simulink model "Aero_UltraStick25e"  (R2016b)
settings: Solver=VariableStepAuto  StartTime=0.0  StopTime=10.0  RelTol=1e-3
undefined symbols (not defined in the file or in its folder): AC
libraries: simulink x1
(part 1 of 2)
settings Model: Creator=UAVLAB  LastModifiedBy=UAVLAB

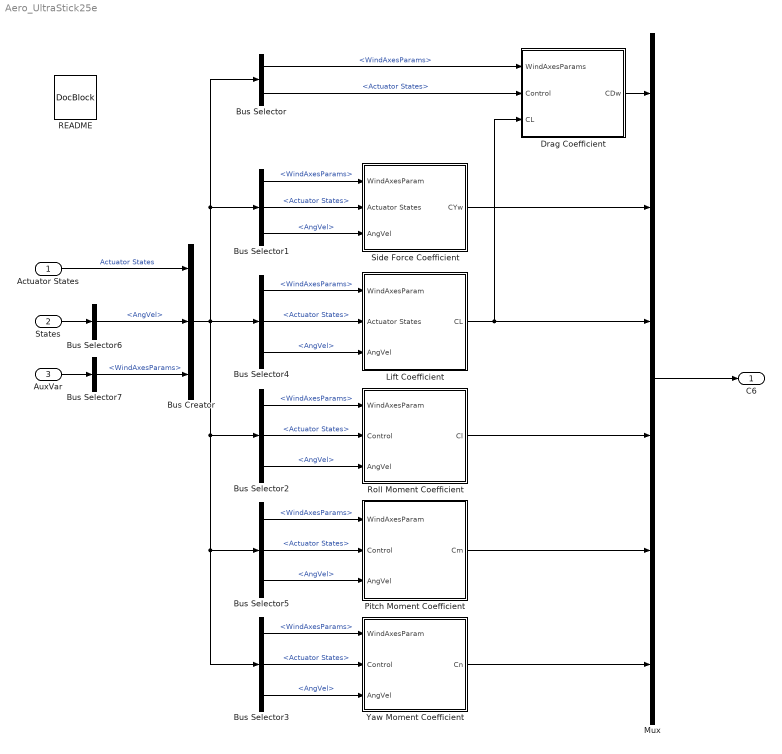
== system Aero_UltraStick25e ==
  Actuator States : Inport  OutDataTypeStr=Bus: Actuators
  States : Inport  Port=2  OutDataTypeStr=Bus: RigidStates
  AuxVar : Inport  Port=3  OutDataTypeStr=Bus: AuxVar
  Bus Creator : BusCreator  Inputs=3
  Bus Selector : BusSelector  OutputSignals=WindAxesParams,Actuator States
  Bus Selector{1..5} (5 alike) : BusSelector  OutputSignals=WindAxesParams,Actuator States,AngVel
  Bus Selector6 : BusSelector  OutputSignals=AngVel
  Bus Selector7 : BusSelector  OutputSignals=WindAxesParams
  Drag Coefficient : Subsystem
  Lift Coefficient : Subsystem
  Mux : Mux  Inputs=6
  Pitch Moment Coefficient : Subsystem
  README : simulink/Model-Wide Utilities/DocBlock  DocumentType=Text
      content=|
      | Ultrastick Aerodynamic Model
      |
      | This block models the Ultrastick aerodynamics using a linear derivatives.
      | The force coefficients are in the wind axes, but the moment coefficients
      | are in body axes, so the six coefficients are CL, CDw, CYw, Cl, Cm, Cn.
      | See Klein, Morelli, Aircraft System Identification, pg 41. Thus in the
      | Aero lib, the force and moment transformation block must be set as though
      | outgoing moment coefficients are in wind axes so no transformation is
      | applied.
      |
      | The derivatives are stored in the aircraft configuration data structure
      | (AC). They are loaded into AC.Aero when 'Ulstrastick' is selected with
      | UAV_config.m.  The derivatives themselves are stored in
      | Ultrastick_config.m. An example is the derivatives for CL:
      |
      | >>  AC.Aero.CL
      |
      | ans =
      |
      |         zero: 0.1086
      |        alpha: 4.5800
      |        dflap: 0.7400
      |        delev: 0.0983
      |     alphadot: 1.9724
      |            q: 6.1639
      |         minD: 0.2300
      |
      | The majority of the derivatives have been indentified from flight test
      | data. The drag model was derived from first principles.
  Roll Moment Coefficient : Subsystem
  Side Force Coefficient : Subsystem
  Yaw Moment Coefficient : Subsystem
  C6 : Outport
  wires:
  Bus Selector/2 -> Drag Coefficient/2(Control)  "<Actuator States>"
  Bus Selector5/3 -> Pitch Moment Coefficient/3(AngVel)  "<AngVel>"
  Bus Selector5/2 -> Pitch Moment Coefficient/2(Control)  "<Actuator States>"
  Bus Selector5/1 -> Pitch Moment Coefficient/1(WindAxesParam)  "<WindAxesParams>"
  Bus Selector4/3 -> Lift Coefficient/3(AngVel)  "<AngVel>"
  Bus Selector4/2 -> Lift Coefficient/2(Actuator States)  "<Actuator States>"
  Bus Selector4/1 -> Lift Coefficient/1(WindAxesParam)  "<WindAxesParams>"
  Bus Selector3/3 -> Yaw Moment Coefficient/3(AngVel)  "<AngVel>"
  Bus Selector3/2 -> Yaw Moment Coefficient/2(Control)  "<Actuator States>"
  Bus Selector3/1 -> Yaw Moment Coefficient/1(WindAxesParam)  "<WindAxesParams>"
  Bus Selector2/3 -> Roll Moment Coefficient/3(AngVel)  "<AngVel>"
  Bus Selector2/2 -> Roll Moment Coefficient/2(Control)  "<Actuator States>"
  Bus Selector2/1 -> Roll Moment Coefficient/1(WindAxesParam)  "<WindAxesParams>"
  Bus Selector1/3 -> Side Force Coefficient/3(AngVel)  "<AngVel>"
  Bus Selector1/2 -> Side Force Coefficient/2(Actuator States)  "<Actuator States>"
  Bus Selector1/1 -> Side Force Coefficient/1(WindAxesParam)  "<WindAxesParams>"
  Bus Creator/1 -> Bus Selector1/1, Bus Selector/1, Bus Selector4/1, Bus Selector5/1, Bus Selector3/1, Bus Selector2/1
  Mux/1 -> C6/1
  Yaw Moment Coefficient/1(Cn) -> Mux/6
  Pitch Moment Coefficient/1(Cm) -> Mux/5
  Roll Moment Coefficient/1(Cl) -> Mux/4
  Side Force Coefficient/1(CYw) -> Mux/2
  Drag Coefficient/1(CDw) -> Mux/1
  States/1 -> Bus Selector6/1
  Bus Selector6/1 -> Bus Creator/2  "<AngVel>"
  Lift Coefficient/1(CL) -> Mux/3, Drag Coefficient/3(CL)
  AuxVar/1 -> Bus Selector7/1
  Bus Selector7/1 -> Bus Creator/3  "<WindAxesParams>"
  Actuator States/1 -> Bus Creator/1  "Actuator States"
  Bus Selector/1 -> Drag Coefficient/1(WindAxesParams)  "<WindAxesParams>"

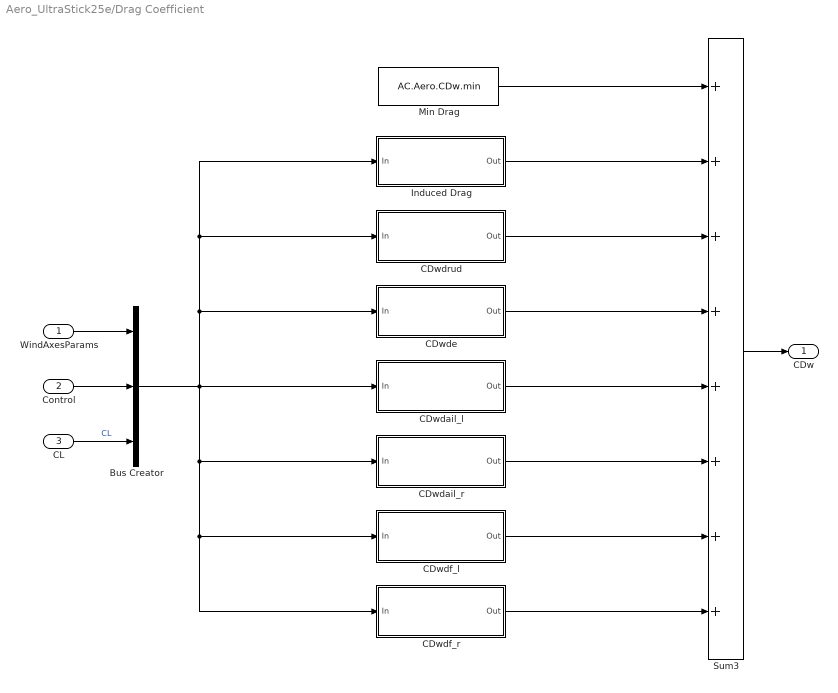
== system Aero_UltraStick25e/Drag Coefficient ==
  WindAxesParams : Inport
  Control : Inport  Port=2
  CL : Inport  Port=3
  Bus Creator : BusCreator  Inputs=3
  CDwdail_l : Subsystem
  CDwdail_r : Subsystem
  CDwde : Subsystem
  CDwdf_l : Subsystem
  CDwdf_r : Subsystem
  CDwdrud : Subsystem
  Induced Drag : Subsystem
  Min Drag : Constant  Value=AC.Aero.CDw.min
  Sum3 : Sum  Inputs=++++++++  SaturateOnIntegerOverflow=on  InputSameDT=on  OutDataTypeStr=Inherit: Same as first input
  CDw : Outport
  wires:
  Min Drag/1 -> Sum3/1
  CDwdrud/1(Out) -> Sum3/3
  CDwde/1(Out) -> Sum3/4
  CDwdail_l/1(Out) -> Sum3/5
  CDwdail_r/1(Out) -> Sum3/6
  CDwdf_l/1(Out) -> Sum3/7
  CDwdf_r/1(Out) -> Sum3/8
  Sum3/1 -> CDw/1
  Bus Creator/1 -> CDwdail_l/1(In), CDwdrud/1(In), Induced Drag/1(In), CDwde/1(In), CDwdail_r/1(In), CDwdf_l/1(In), CDwdf_r/1(In)
  Induced Drag/1(Out) -> Sum3/2
  WindAxesParams/1 -> Bus Creator/1
  Control/1 -> Bus Creator/2
  CL/1 -> Bus Creator/3  "CL"

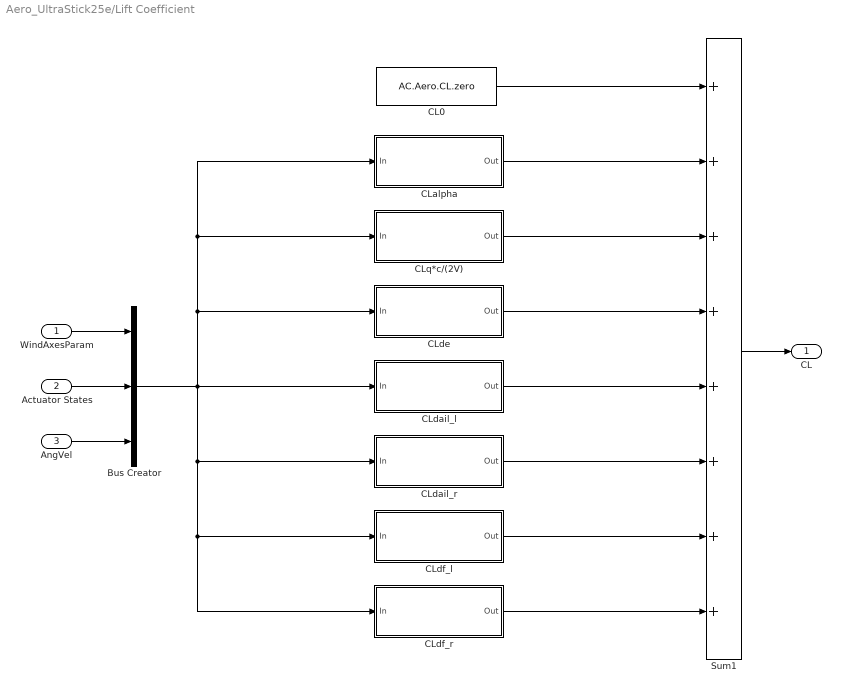
== system Aero_UltraStick25e/Lift Coefficient ==
  WindAxesParam : Inport
  Actuator States : Inport  Port=2  OutDataTypeStr=Bus: Actuators
  AngVel : Inport  Port=3
  Bus Creator : BusCreator  Inputs=3
  CL0 : Constant  Value=AC.Aero.CL.zero
  CLalpha : Subsystem
  CLdail_l : Subsystem
  CLdail_r : Subsystem
  CLde : Subsystem
  CLdf_l : Subsystem
  CLdf_r : Subsystem
  CLq*c/(2V) : Subsystem
  Sum1 : Sum  Inputs=++++++++  SaturateOnIntegerOverflow=on  InputSameDT=on  OutDataTypeStr=Inherit: Same as first input
  CL : Outport
  wires:
  WindAxesParam/1 -> Bus Creator/1
  Actuator States/1 -> Bus Creator/2
  AngVel/1 -> Bus Creator/3
  Bus Creator/1 -> CLdail_l/1(In), CLalpha/1(In), CLq*c/(2V)/1(In), CLde/1(In), CLdail_r/1(In), CLdf_l/1(In), CLdf_r/1(In)
  CLalpha/1(Out) -> Sum1/2
  CL0/1 -> Sum1/1
  CLq*c/(2V)/1(Out) -> Sum1/3
  CLde/1(Out) -> Sum1/4
  CLdail_l/1(Out) -> Sum1/5
  CLdail_r/1(Out) -> Sum1/6
  CLdf_l/1(Out) -> Sum1/7
  CLdf_r/1(Out) -> Sum1/8
  Sum1/1 -> CL/1

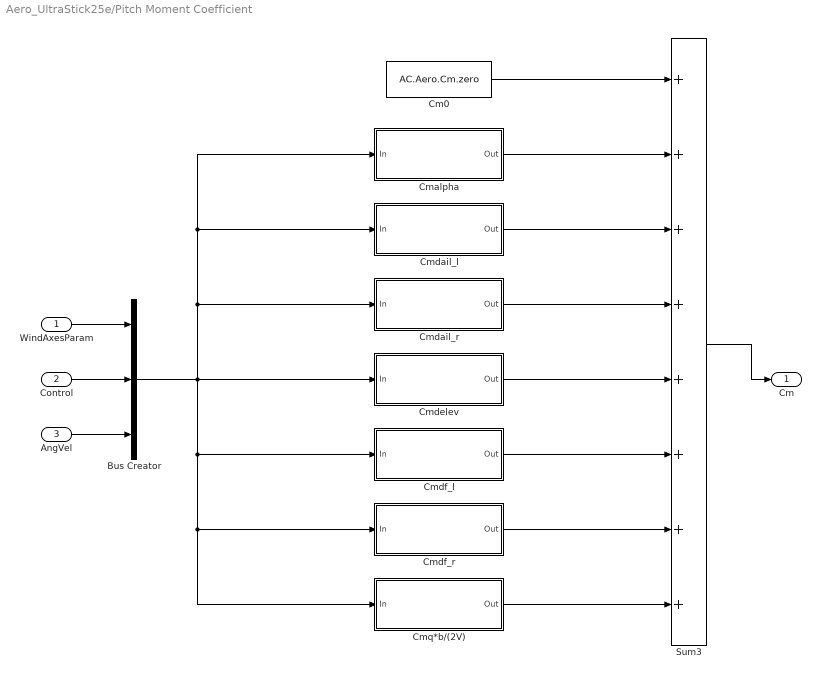
== system Aero_UltraStick25e/Pitch Moment Coefficient ==
  WindAxesParam : Inport
  Control : Inport  Port=2
  AngVel : Inport  Port=3
  Bus Creator : BusCreator  Inputs=3
  Cm0 : Constant  Value=AC.Aero.Cm.zero
  Cmalpha : Subsystem
  Cmdail_l : Subsystem
  Cmdail_r : Subsystem
  Cmdelev : Subsystem
  Cmdf_l : Subsystem
  Cmdf_r : Subsystem
  Cmq*b/(2V) : Subsystem
  Sum3 : Sum  Inputs=++++++++  SaturateOnIntegerOverflow=on  InputSameDT=on  OutDataTypeStr=Inherit: Same as first input
  Cm : Outport
  wires:
  WindAxesParam/1 -> Bus Creator/1
  Control/1 -> Bus Creator/2
  AngVel/1 -> Bus Creator/3
  Bus Creator/1 -> Cmdf_l/1(In), Cmdf_r/1(In), Cmq*b/(2V)/1(In), Cmdelev/1(In), Cmdail_l/1(In), Cmalpha/1(In), Cmdail_r/1(In)
  Cmq*b/(2V)/1(Out) -> Sum3/8
  Cmdf_r/1(Out) -> Sum3/7
  Cmdf_l/1(Out) -> Sum3/6
  Cmdelev/1(Out) -> Sum3/5
  Cmdail_l/1(Out) -> Sum3/3
  Cmdail_r/1(Out) -> Sum3/4
  Cmalpha/1(Out) -> Sum3/2
  Cm0/1 -> Sum3/1
  Sum3/1 -> Cm/1

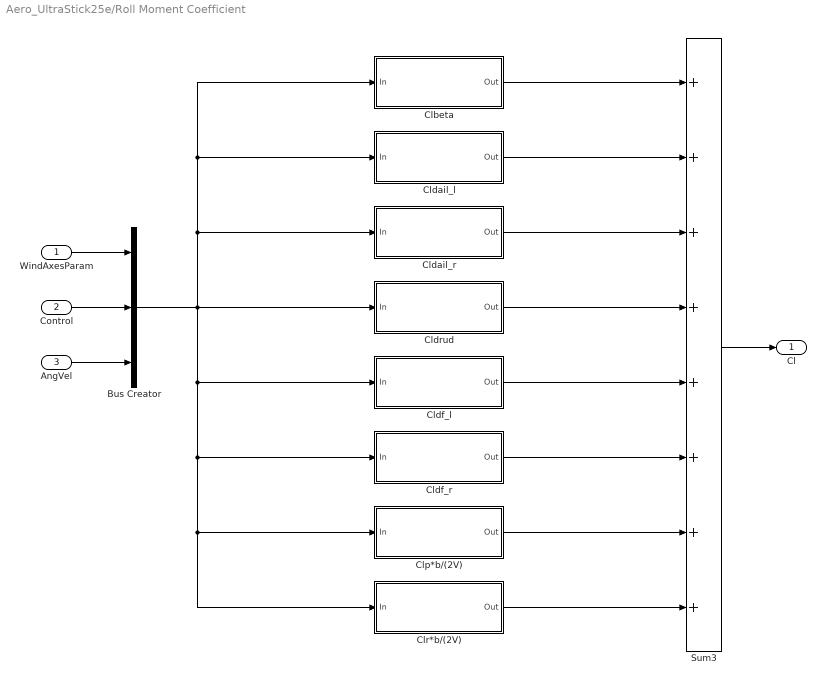
== system Aero_UltraStick25e/Roll Moment Coefficient ==
  WindAxesParam : Inport
  Control : Inport  Port=2
  AngVel : Inport  Port=3
  Bus Creator : BusCreator  Inputs=3
  Clbeta : Subsystem
  Cldail_l : Subsystem
  Cldail_r : Subsystem
  Cldf_l : Subsystem
  Cldf_r : Subsystem
  Cldrud : Subsystem
  Clp*b/(2V) : Subsystem
  Clr*b/(2V) : Subsystem
  Sum3 : Sum  Inputs=++++++++  SaturateOnIntegerOverflow=on  InputSameDT=on  OutDataTypeStr=Inherit: Same as first input
  Cl : Outport
  wires:
  WindAxesParam/1 -> Bus Creator/1
  Control/1 -> Bus Creator/2
  AngVel/1 -> Bus Creator/3
  Sum3/1 -> Cl/1
  Clbeta/1(Out) -> Sum3/1
  Cldail_r/1(Out) -> Sum3/3
  Cldail_l/1(Out) -> Sum3/2
  Clr*b/(2V)/1(Out) -> Sum3/8
  Clp*b/(2V)/1(Out) -> Sum3/7
  Bus Creator/1 -> Cldf_l/1(In), Cldf_r/1(In), Clr*b/(2V)/1(In), Clp*b/(2V)/1(In), Cldrud/1(In), Cldail_l/1(In), Clbeta/1(In), Cldail_r/1(In)
  Cldf_r/1(Out) -> Sum3/6
  Cldf_l/1(Out) -> Sum3/5
  Cldrud/1(Out) -> Sum3/4

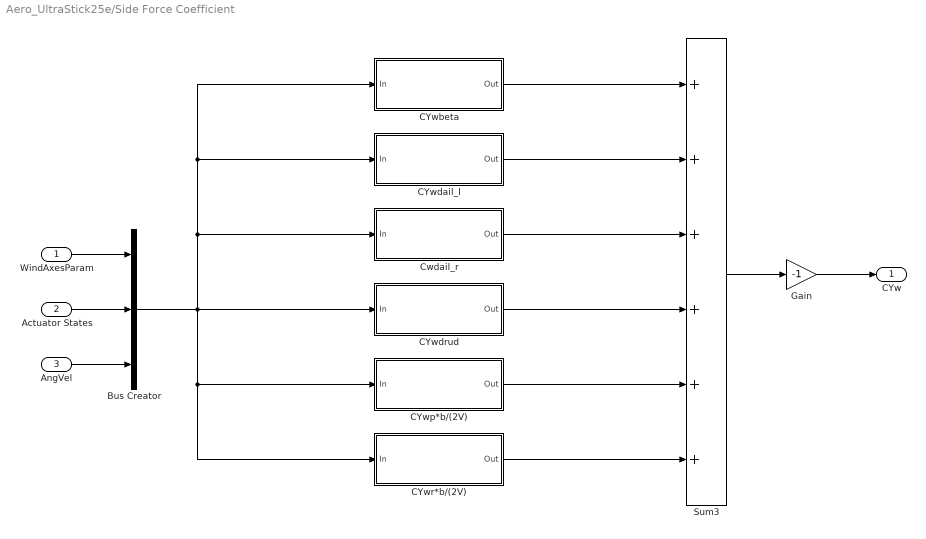
== system Aero_UltraStick25e/Side Force Coefficient ==
  WindAxesParam : Inport
  Actuator States : Inport  Port=2  OutDataTypeStr=Bus: Actuators
  AngVel : Inport  Port=3
  Bus Creator : BusCreator  Inputs=3
  CYwbeta : Subsystem
  CYwdail_l : Subsystem
  CYwdrud : Subsystem
  CYwp*b/(2V) : Subsystem
  CYwr*b/(2V) : Subsystem
  Cwdail_r : Subsystem
  Gain : Gain  Gain=-1
  Sum3 : Sum  Inputs=++++++  SaturateOnIntegerOverflow=on  InputSameDT=on  OutDataTypeStr=Inherit: Same as first input
  CYw : Outport
  wires:
  WindAxesParam/1 -> Bus Creator/1
  Actuator States/1 -> Bus Creator/2
  AngVel/1 -> Bus Creator/3
  Bus Creator/1 -> CYwr*b/(2V)/1(In), CYwp*b/(2V)/1(In), CYwdrud/1(In), CYwdail_l/1(In), CYwbeta/1(In), Cwdail_r/1(In)
  Sum3/1 -> Gain/1
  Gain/1 -> CYw/1
  CYwbeta/1(Out) -> Sum3/1
  CYwr*b/(2V)/1(Out) -> Sum3/6
  CYwp*b/(2V)/1(Out) -> Sum3/5
  CYwdrud/1(Out) -> Sum3/4
  Cwdail_r/1(Out) -> Sum3/3
  CYwdail_l/1(Out) -> Sum3/2

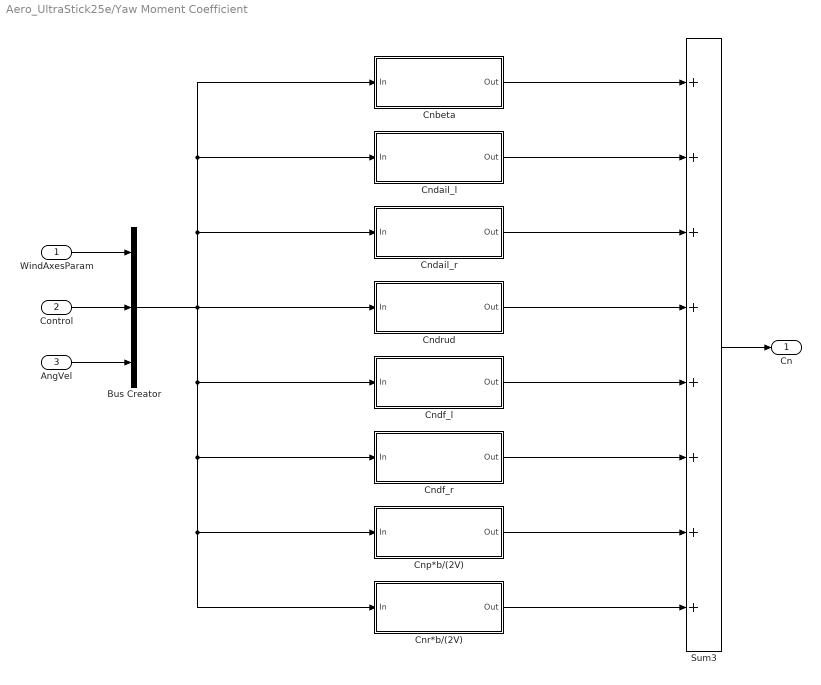
== system Aero_UltraStick25e/Yaw Moment Coefficient ==
  WindAxesParam : Inport
  Control : Inport  Port=2
  AngVel : Inport  Port=3
  Bus Creator : BusCreator  Inputs=3
  Cnbeta : Subsystem
  Cndail_l : Subsystem
  Cndail_r : Subsystem
  Cndf_l : Subsystem
  Cndf_r : Subsystem
  Cndrud : Subsystem
  Cnp*b/(2V) : Subsystem
  Cnr*b/(2V) : Subsystem
  Sum3 : Sum  Inputs=++++++++  SaturateOnIntegerOverflow=on  InputSameDT=on  OutDataTypeStr=Inherit: Same as first input
  Cn : Outport
  wires:
  WindAxesParam/1 -> Bus Creator/1
  Control/1 -> Bus Creator/2
  AngVel/1 -> Bus Creator/3
  Cnbeta/1(Out) -> Sum3/1
  Cndail_r/1(Out) -> Sum3/3
  Cndail_l/1(Out) -> Sum3/2
  Cnr*b/(2V)/1(Out) -> Sum3/8
  Cnp*b/(2V)/1(Out) -> Sum3/7
  Bus Creator/1 -> Cndf_l/1(In), Cndf_r/1(In), Cnr*b/(2V)/1(In), Cnp*b/(2V)/1(In), Cndrud/1(In), Cndail_l/1(In), Cnbeta/1(In), Cndail_r/1(In)
  Cndf_r/1(Out) -> Sum3/6
  Cndf_l/1(Out) -> Sum3/5
  Cndrud/1(Out) -> Sum3/4
  Sum3/1 -> Cn/1

== system Aero_UltraStick25e/Drag Coefficient/CDwdail_l ==
  In : Inport
  Abs : Abs  SaturateOnIntegerOverflow=on
  Bus Selector4 : BusSelector  OutputSignals=Actuator States.CtrlSurf.l_aileron_rad,WindAxesParams.alpha_rad,WindAxesParams.beta_rad
  CDwdail_l : Product
  CDwdail_l Lookup : Interpolation_n-D  Table=AC.Aero.CDw.dail_dat.data  InternalRulePriority=Speed
  Prelookup Alpha : PreLookup  BreakpointsData=AC.Aero.CL.alpha_dat.alpha  ExtrapMethod=Linear
  Prelookup Beta : PreLookup  BreakpointsData=AC.Aero.CL.alpha_dat.beta  ExtrapMethod=Linear
  Out : Outport
  wires:
  CDwdail_l/1 -> Abs/1
  CDwdail_l Lookup/1 -> CDwdail_l/2
  Prelookup Alpha/2 -> CDwdail_l Lookup/2
  Bus Selector4/2 -> Prelookup Alpha/1  "<alpha_rad>"
  Bus Selector4/3 -> Prelookup Beta/1  "<beta_rad>"
  Prelookup Alpha/1 -> CDwdail_l Lookup/1
  Prelookup Beta/2 -> CDwdail_l Lookup/4
  Prelookup Beta/1 -> CDwdail_l Lookup/3
  In/1 -> Bus Selector4/1
  Bus Selector4/1 -> CDwdail_l/1  "<l_aileron_rad>"
  Abs/1 -> Out/1

== system Aero_UltraStick25e/Drag Coefficient/CDwdail_r ==
  In : Inport
  Abs : Abs  SaturateOnIntegerOverflow=on
  Bus Selector4 : BusSelector  OutputSignals=Actuator States.CtrlSurf.r_aileron_rad,WindAxesParams.alpha_rad,WindAxesParams.beta_rad
  CDwdail_r : Product
  CDwdail_r Lookup : Interpolation_n-D  Table=AC.Aero.CDw.dail_dat.data  InternalRulePriority=Speed
  Prelookup Alpha : PreLookup  BreakpointsData=AC.Aero.CL.alpha_dat.alpha  ExtrapMethod=Linear
  Prelookup Beta : PreLookup  BreakpointsData=AC.Aero.CL.alpha_dat.beta  ExtrapMethod=Linear
  Out : Outport
  wires:
  CDwdail_r/1 -> Abs/1
  CDwdail_r Lookup/1 -> CDwdail_r/2
  Prelookup Alpha/2 -> CDwdail_r Lookup/2
  Bus Selector4/2 -> Prelookup Alpha/1  "<alpha_rad>"
  Bus Selector4/3 -> Prelookup Beta/1  "<beta_rad>"
  Prelookup Alpha/1 -> CDwdail_r Lookup/1
  Prelookup Beta/2 -> CDwdail_r Lookup/4
  Prelookup Beta/1 -> CDwdail_r Lookup/3
  In/1 -> Bus Selector4/1
  Bus Selector4/1 -> CDwdail_r/1  "<r_aileron_rad>"
  Abs/1 -> Out/1

== system Aero_UltraStick25e/Drag Coefficient/CDwde ==
  In : Inport
  Abs2 : Abs  SaturateOnIntegerOverflow=on
  Bus Selector4 : BusSelector  OutputSignals=Actuator States.CtrlSurf.elevator_rad,WindAxesParams.alpha_rad,WindAxesParams.beta_rad
  CDwde : Product
  CDwde Lookup : Interpolation_n-D  Table=AC.Aero.CDw.dele_dat.data  InternalRulePriority=Speed
  Prelookup Alpha : PreLookup  BreakpointsData=AC.Aero.CL.alpha_dat.alpha  ExtrapMethod=Linear
  Prelookup Beta : PreLookup  BreakpointsData=AC.Aero.CL.alpha_dat.beta  ExtrapMethod=Linear
  Out : Outport
  wires:
  CDwde/1 -> Abs2/1
  CDwde Lookup/1 -> CDwde/2
  Prelookup Alpha/2 -> CDwde Lookup/2
  Bus Selector4/2 -> Prelookup Alpha/1  "<alpha_rad>"
  Bus Selector4/3 -> Prelookup Beta/1  "<beta_rad>"
  Prelookup Alpha/1 -> CDwde Lookup/1
  Prelookup Beta/2 -> CDwde Lookup/4
  Prelookup Beta/1 -> CDwde Lookup/3
  In/1 -> Bus Selector4/1
  Bus Selector4/1 -> CDwde/1  "<elevator_rad>"
  Abs2/1 -> Out/1

== system Aero_UltraStick25e/Drag Coefficient/CDwdf_l ==
  In : Inport
  Abs : Abs  SaturateOnIntegerOverflow=on
  Bus Selector4 : BusSelector  OutputSignals=Actuator States.CtrlSurf.l_flap_rad,WindAxesParams.alpha_rad,WindAxesParams.beta_rad
  CDwdf_l : Product
  CDwdf_l Lookup : Interpolation_n-D  Table=AC.Aero.CDw.dflap_dat.data  InternalRulePriority=Speed
  Prelookup Alpha : PreLookup  BreakpointsData=AC.Aero.CL.alpha_dat.alpha  ExtrapMethod=Linear
  Prelookup Beta : PreLookup  BreakpointsData=AC.Aero.CL.alpha_dat.beta  ExtrapMethod=Linear
  Out : Outport
  wires:
  CDwdf_l/1 -> Abs/1
  CDwdf_l Lookup/1 -> CDwdf_l/2
  Prelookup Alpha/2 -> CDwdf_l Lookup/2
  Bus Selector4/2 -> Prelookup Alpha/1  "<alpha_rad>"
  Bus Selector4/3 -> Prelookup Beta/1  "<beta_rad>"
  Prelookup Alpha/1 -> CDwdf_l Lookup/1
  Prelookup Beta/2 -> CDwdf_l Lookup/4
  Prelookup Beta/1 -> CDwdf_l Lookup/3
  In/1 -> Bus Selector4/1
  Bus Selector4/1 -> CDwdf_l/1  "<l_flap_rad>"
  Abs/1 -> Out/1

== system Aero_UltraStick25e/Drag Coefficient/CDwdf_r ==
  In : Inport
  Abs : Abs  SaturateOnIntegerOverflow=on
  Bus Selector4 : BusSelector  OutputSignals=Actuator States.CtrlSurf.r_flap_rad,WindAxesParams.alpha_rad,WindAxesParams.beta_rad
  CDwdf_r : Product
  CDwdf_r Lookup : Interpolation_n-D  Table=AC.Aero.CDw.dflap_dat.data  InternalRulePriority=Speed
  Prelookup Alpha : PreLookup  BreakpointsData=AC.Aero.CL.alpha_dat.alpha  ExtrapMethod=Linear
  Prelookup Beta : PreLookup  BreakpointsData=AC.Aero.CL.alpha_dat.beta  ExtrapMethod=Linear
  Out : Outport
  wires:
  CDwdf_r/1 -> Abs/1
  CDwdf_r Lookup/1 -> CDwdf_r/2
  Prelookup Alpha/2 -> CDwdf_r Lookup/2
  Bus Selector4/2 -> Prelookup Alpha/1  "<alpha_rad>"
  Bus Selector4/3 -> Prelookup Beta/1  "<beta_rad>"
  Prelookup Alpha/1 -> CDwdf_r Lookup/1
  Prelookup Beta/2 -> CDwdf_r Lookup/4
  Prelookup Beta/1 -> CDwdf_r Lookup/3
  In/1 -> Bus Selector4/1
  Bus Selector4/1 -> CDwdf_r/1  "<r_flap_rad>"
  Abs/1 -> Out/1

== system Aero_UltraStick25e/Drag Coefficient/CDwdrud ==
  In : Inport
  Abs : Abs  SaturateOnIntegerOverflow=on
  Bus Selector4 : BusSelector  OutputSignals=Actuator States.CtrlSurf.rudder_rad,WindAxesParams.alpha_rad,WindAxesParams.beta_rad
  CDwdrud : Product
  CDwdrud Lookup : Interpolation_n-D  Table=AC.Aero.CDw.drud_dat.data  InternalRulePriority=Speed
  Prelookup Alpha : PreLookup  BreakpointsData=AC.Aero.CL.alpha_dat.alpha  ExtrapMethod=Linear
  Prelookup Beta : PreLookup  BreakpointsData=AC.Aero.CL.alpha_dat.beta  ExtrapMethod=Linear
  Out : Outport
  wires:
  CDwdrud/1 -> Abs/1
  CDwdrud Lookup/1 -> CDwdrud/2
  Prelookup Alpha/2 -> CDwdrud Lookup/2
  Bus Selector4/2 -> Prelookup Alpha/1  "<alpha_rad>"
  Bus Selector4/3 -> Prelookup Beta/1  "<beta_rad>"
  Prelookup Alpha/1 -> CDwdrud Lookup/1
  Prelookup Beta/2 -> CDwdrud Lookup/4
  Prelookup Beta/1 -> CDwdrud Lookup/3
  In/1 -> Bus Selector4/1
  Bus Selector4/1 -> CDwdrud/1  "<rudder_rad>"
  Abs/1 -> Out/1

== system Aero_UltraStick25e/Drag Coefficient/Induced Drag ==
  In : Inport
  Bus Selector : BusSelector  OutputSignals=CL
  CL min drag : Constant  Value=AC.Aero.CL.minD
  CL^1 : Math  Operator=square  SaturateOnIntegerOverflow=on
  Induced Drag : Gain  Gain=1/(pi*AC.Geometry.b^2/AC.Geometry.S*AC.Aero.CDw.osw);  SaturateOnIntegerOverflow=on  OutDataTypeStr=Inherit: Same as input  ParamDataTypeStr=Inherit: Same as input
  Sum4 : Sum  Inputs=|+-  SaturateOnIntegerOverflow=on  InputSameDT=on  OutDataTypeStr=Inherit: Same as first input
  Out : Outport
  wires:
  In/1 -> Bus Selector/1
  Sum4/1 -> CL^1/1
  CL^1/1 -> Induced Drag/1
  CL min drag/1 -> Sum4/2
  Induced Drag/1 -> Out/1
  Bus Selector/1 -> Sum4/1  "<CL>"

== system Aero_UltraStick25e/Lift Coefficient/CLalpha ==
  In : Inport
  Bus Selector4 : BusSelector  OutputSignals=WindAxesParams.alpha_rad,WindAxesParams.beta_rad
  CLalpha : Product
  CLalpha Lookup : Interpolation_n-D  Table=AC.Aero.CL.alpha_dat.data  InternalRulePriority=Speed
  Prelookup Alpha : PreLookup  BreakpointsData=AC.Aero.CL.alpha_dat.alpha  ExtrapMethod=Linear
  Prelookup Beta : PreLookup  BreakpointsData=AC.Aero.CL.alpha_dat.beta  ExtrapMethod=Linear
  Out : Outport
  wires:
  In/1 -> Bus Selector4/1
  Prelookup Beta/1 -> CLalpha Lookup/3
  Prelookup Beta/2 -> CLalpha Lookup/4
  Prelookup Alpha/1 -> CLalpha Lookup/1
  Bus Selector4/2 -> Prelookup Beta/1  "<beta_rad>"
  Bus Selector4/1 -> CLalpha/1, Prelookup Alpha/1  "<alpha_rad>"
  Prelookup Alpha/2 -> CLalpha Lookup/2
  CLalpha Lookup/1 -> CLalpha/2
  CLalpha/1 -> Out/1

== system Aero_UltraStick25e/Lift Coefficient/CLdail_l ==
  In : Inport
  Bus Selector4 : BusSelector  OutputSignals=Actuator States.CtrlSurf.l_aileron_rad,WindAxesParams.alpha_rad,WindAxesParams.beta_rad
  CLdail_l : Product
  CLdail_l Lookup : Interpolation_n-D  Table=AC.Aero.CL.dail_dat.data  InternalRulePriority=Speed
  Prelookup Alpha : PreLookup  BreakpointsData=AC.Aero.CL.alpha_dat.alpha  ExtrapMethod=Linear
  Prelookup Beta : PreLookup  BreakpointsData=AC.Aero.CL.alpha_dat.beta  ExtrapMethod=Linear
  Out : Outport
  wires:
  CLdail_l/1 -> Out/1
  CLdail_l Lookup/1 -> CLdail_l/2
  Prelookup Alpha/2 -> CLdail_l Lookup/2
  Bus Selector4/2 -> Prelookup Alpha/1  "<alpha_rad>"
  Bus Selector4/3 -> Prelookup Beta/1  "<beta_rad>"
  Prelookup Alpha/1 -> CLdail_l Lookup/1
  Prelookup Beta/2 -> CLdail_l Lookup/4
  Prelookup Beta/1 -> CLdail_l Lookup/3
  In/1 -> Bus Selector4/1
  Bus Selector4/1 -> CLdail_l/1  "<l_aileron_rad>"

== system Aero_UltraStick25e/Lift Coefficient/CLdail_r ==
  In : Inport
  Bus Selector4 : BusSelector  OutputSignals=Actuator States.CtrlSurf.r_aileron_rad,WindAxesParams.alpha_rad,WindAxesParams.beta_rad
  CLdail_r : Product
  CLdail_r Lookup : Interpolation_n-D  Table=AC.Aero.CL.dail_dat.data  InternalRulePriority=Speed
  Prelookup Alpha : PreLookup  BreakpointsData=AC.Aero.CL.alpha_dat.alpha  ExtrapMethod=Linear
  Prelookup Beta : PreLookup  BreakpointsData=AC.Aero.CL.alpha_dat.beta  ExtrapMethod=Linear
  Out : Outport
  wires:
  CLdail_r/1 -> Out/1
  CLdail_r Lookup/1 -> CLdail_r/2
  Prelookup Alpha/2 -> CLdail_r Lookup/2
  Bus Selector4/2 -> Prelookup Alpha/1  "<alpha_rad>"
  Bus Selector4/3 -> Prelookup Beta/1  "<beta_rad>"
  Prelookup Alpha/1 -> CLdail_r Lookup/1
  Prelookup Beta/2 -> CLdail_r Lookup/4
  Prelookup Beta/1 -> CLdail_r Lookup/3
  In/1 -> Bus Selector4/1
  Bus Selector4/1 -> CLdail_r/1  "<r_aileron_rad>"

== system Aero_UltraStick25e/Lift Coefficient/CLde ==
  In : Inport
  Bus Selector4 : BusSelector  OutputSignals=Actuator States.CtrlSurf.elevator_rad,WindAxesParams.alpha_rad,WindAxesParams.beta_rad
  CLde : Product
  CLde Lookup : Interpolation_n-D  Table=AC.Aero.CL.dele_dat.data  InternalRulePriority=Speed
  Prelookup Alpha : PreLookup  BreakpointsData=AC.Aero.CL.alpha_dat.alpha  ExtrapMethod=Linear
  Prelookup Beta : PreLookup  BreakpointsData=AC.Aero.CL.alpha_dat.beta  ExtrapMethod=Linear
  Out : Outport
  wires:
  CLde/1 -> Out/1
  CLde Lookup/1 -> CLde/2
  Prelookup Alpha/2 -> CLde Lookup/2
  Bus Selector4/2 -> Prelookup Alpha/1  "<alpha_rad>"
  Bus Selector4/3 -> Prelookup Beta/1  "<beta_rad>"
  Prelookup Alpha/1 -> CLde Lookup/1
  Prelookup Beta/2 -> CLde Lookup/4
  Prelookup Beta/1 -> CLde Lookup/3
  In/1 -> Bus Selector4/1
  Bus Selector4/1 -> CLde/1  "<elevator_rad>"

== system Aero_UltraStick25e/Lift Coefficient/CLdf_l ==
  In : Inport
  Bus Selector4 : BusSelector  OutputSignals=Actuator States.CtrlSurf.l_flap_rad,WindAxesParams.alpha_rad,WindAxesParams.beta_rad
  CLdf_l : Product
  CLdf_l Lookup : Interpolation_n-D  Table=AC.Aero.CL.dflap_dat.data  InternalRulePriority=Speed
  Prelookup Alpha : PreLookup  BreakpointsData=AC.Aero.CL.alpha_dat.alpha  ExtrapMethod=Linear
  Prelookup Beta : PreLookup  BreakpointsData=AC.Aero.CL.alpha_dat.beta  ExtrapMethod=Linear
  Out : Outport
  wires:
  CLdf_l/1 -> Out/1
  CLdf_l Lookup/1 -> CLdf_l/2
  Prelookup Alpha/2 -> CLdf_l Lookup/2
  Bus Selector4/2 -> Prelookup Alpha/1  "<alpha_rad>"
  Bus Selector4/3 -> Prelookup Beta/1  "<beta_rad>"
  Prelookup Alpha/1 -> CLdf_l Lookup/1
  Prelookup Beta/2 -> CLdf_l Lookup/4
  Prelookup Beta/1 -> CLdf_l Lookup/3
  In/1 -> Bus Selector4/1
  Bus Selector4/1 -> CLdf_l/1  "<l_flap_rad>"

== system Aero_UltraStick25e/Lift Coefficient/CLdf_r ==
  In : Inport
  Bus Selector4 : BusSelector  OutputSignals=Actuator States.CtrlSurf.r_flap_rad,WindAxesParams.alpha_rad,WindAxesParams.beta_rad
  CLdf_r : Product
  CLdf_r Lookup : Interpolation_n-D  Table=AC.Aero.CL.dflap_dat.data  InternalRulePriority=Speed
  Prelookup Alpha : PreLookup  BreakpointsData=AC.Aero.CL.alpha_dat.alpha  ExtrapMethod=Linear
  Prelookup Beta : PreLookup  BreakpointsData=AC.Aero.CL.alpha_dat.beta  ExtrapMethod=Linear
  Out : Outport
  wires:
  CLdf_r/1 -> Out/1
  CLdf_r Lookup/1 -> CLdf_r/2
  Prelookup Alpha/2 -> CLdf_r Lookup/2
  Bus Selector4/2 -> Prelookup Alpha/1  "<alpha_rad>"
  Bus Selector4/3 -> Prelookup Beta/1  "<beta_rad>"
  Prelookup Alpha/1 -> CLdf_r Lookup/1
  Prelookup Beta/2 -> CLdf_r Lookup/4
  Prelookup Beta/1 -> CLdf_r Lookup/3
  In/1 -> Bus Selector4/1
  Bus Selector4/1 -> CLdf_r/1  "<r_flap_rad>"

== system Aero_UltraStick25e/Lift Coefficient/CLq*c//(2V) ==
  In : Inport
  2 : Gain  Gain=2  SaturateOnIntegerOverflow=on  OutDataTypeStr=Inherit: Same as input  ParamDataTypeStr=Inherit: Same as input
  Bus Selector : BusSelector  OutputSignals=WindAxesParams.Vs_mps
  CL*c/(2V) : Product  Inputs=**/  SaturateOnIntegerOverflow=on  InputSameDT=on  OutDataTypeStr=Inherit: Same as first input
  CLq : Subsystem
  Wing chord : Constant  Value=AC.Geometry.c
  Out : Outport
  wires:
  CL*c/(2V)/1 -> Out/1
  Wing chord/1 -> CL*c/(2V)/2
  2/1 -> CL*c/(2V)/3
  In/1 -> Bus Selector/1, CLq/1(In)
  Bus Selector/1 -> 2/1  "<Vs_mps>"
  CLq/1(Out) -> CL*c/(2V)/1

== system Aero_UltraStick25e/Pitch Moment Coefficient/Cmalpha ==
  In : Inport
  Bus Selector4 : BusSelector  OutputSignals=WindAxesParams.alpha_rad,WindAxesParams.beta_rad
  Cmalpha : Product
  Cmalpha Lookup : Interpolation_n-D  Table=AC.Aero.Cm.alpha_dat.data  InternalRulePriority=Speed
  Prelookup Alpha : PreLookup  BreakpointsData=AC.Aero.CL.alpha_dat.alpha  ExtrapMethod=Linear
  Prelookup Beta : PreLookup  BreakpointsData=AC.Aero.CL.alpha_dat.beta  ExtrapMethod=Linear
  Out : Outport
  wires:
  In/1 -> Bus Selector4/1
  Prelookup Beta/1 -> Cmalpha Lookup/3
  Prelookup Beta/2 -> Cmalpha Lookup/4
  Prelookup Alpha/1 -> Cmalpha Lookup/1
  Bus Selector4/2 -> Prelookup Beta/1  "<beta_rad>"
  Bus Selector4/1 -> Cmalpha/1, Prelookup Alpha/1  "<alpha_rad>"
  Prelookup Alpha/2 -> Cmalpha Lookup/2
  Cmalpha/1 -> Out/1
  Cmalpha Lookup/1 -> Cmalpha/2

== system Aero_UltraStick25e/Pitch Moment Coefficient/Cmdail_l ==
  In : Inport
  Bus Selector4 : BusSelector  OutputSignals=Actuator States.CtrlSurf.l_aileron_rad,WindAxesParams.alpha_rad,WindAxesParams.beta_rad
  Cmdail_l : Product
  Cmdail_l Lookup : Interpolation_n-D  Table=AC.Aero.Cm.dail_dat.data  InternalRulePriority=Speed
  Prelookup Alpha : PreLookup  BreakpointsData=AC.Aero.CL.alpha_dat.alpha  ExtrapMethod=Linear
  Prelookup Beta : PreLookup  BreakpointsData=AC.Aero.CL.alpha_dat.beta  ExtrapMethod=Linear
  Out : Outport
  wires:
  Cmdail_l Lookup/1 -> Cmdail_l/2
  Prelookup Alpha/2 -> Cmdail_l Lookup/2
  Bus Selector4/2 -> Prelookup Alpha/1  "<alpha_rad>"
  Bus Selector4/3 -> Prelookup Beta/1  "<beta_rad>"
  Prelookup Alpha/1 -> Cmdail_l Lookup/1
  Prelookup Beta/2 -> Cmdail_l Lookup/4
  Prelookup Beta/1 -> Cmdail_l Lookup/3
  In/1 -> Bus Selector4/1
  Bus Selector4/1 -> Cmdail_l/1  "<l_aileron_rad>"
  Cmdail_l/1 -> Out/1

== system Aero_UltraStick25e/Pitch Moment Coefficient/Cmdail_r ==
  In : Inport
  Bus Selector4 : BusSelector  OutputSignals=Actuator States.CtrlSurf.r_aileron_rad,WindAxesParams.alpha_rad,WindAxesParams.beta_rad
  Cmdail_r : Product
  Cmdail_r Lookup : Interpolation_n-D  Table=AC.Aero.Cm.dail_dat.data  InternalRulePriority=Speed
  Prelookup Alpha : PreLookup  BreakpointsData=AC.Aero.CL.alpha_dat.alpha  ExtrapMethod=Linear
  Prelookup Beta : PreLookup  BreakpointsData=AC.Aero.CL.alpha_dat.beta  ExtrapMethod=Linear
  Out : Outport
  wires:
  Cmdail_r/1 -> Out/1
  Cmdail_r Lookup/1 -> Cmdail_r/2
  Prelookup Alpha/2 -> Cmdail_r Lookup/2
  Bus Selector4/2 -> Prelookup Alpha/1  "<alpha_rad>"
  Bus Selector4/3 -> Prelookup Beta/1  "<beta_rad>"
  Prelookup Alpha/1 -> Cmdail_r Lookup/1
  Prelookup Beta/2 -> Cmdail_r Lookup/4
  Prelookup Beta/1 -> Cmdail_r Lookup/3
  In/1 -> Bus Selector4/1
  Bus Selector4/1 -> Cmdail_r/1  "<r_aileron_rad>"

== system Aero_UltraStick25e/Pitch Moment Coefficient/Cmdelev ==
  In : Inport
  Bus Selector4 : BusSelector  OutputSignals=Actuator States.CtrlSurf.elevator_rad,WindAxesParams.alpha_rad,WindAxesParams.beta_rad
  Cmdelev : Product
  Cmdelev Lookup : Interpolation_n-D  Table=AC.Aero.Cm.delev_dat.data  InternalRulePriority=Speed
  Prelookup Alpha : PreLookup  BreakpointsData=AC.Aero.CL.alpha_dat.alpha  ExtrapMethod=Linear
  Prelookup Beta : PreLookup  BreakpointsData=AC.Aero.CL.alpha_dat.beta  ExtrapMethod=Linear
  Out : Outport
  wires:
  Cmdelev Lookup/1 -> Cmdelev/2
  Prelookup Alpha/2 -> Cmdelev Lookup/2
  Bus Selector4/2 -> Prelookup Alpha/1  "<alpha_rad>"
  Bus Selector4/3 -> Prelookup Beta/1  "<beta_rad>"
  Prelookup Alpha/1 -> Cmdelev Lookup/1
  Prelookup Beta/2 -> Cmdelev Lookup/4
  Prelookup Beta/1 -> Cmdelev Lookup/3
  In/1 -> Bus Selector4/1
  Bus Selector4/1 -> Cmdelev/1  "<elevator_rad>"
  Cmdelev/1 -> Out/1

== system Aero_UltraStick25e/Pitch Moment Coefficient/Cmdf_l ==
  In : Inport
  Bus Selector4 : BusSelector  OutputSignals=Actuator States.CtrlSurf.l_flap_rad,WindAxesParams.alpha_rad,WindAxesParams.beta_rad
  Cmdf_l : Product
  Cmdf_l Lookup : Interpolation_n-D  Table=AC.Aero.Cm.dflap_dat.data  InternalRulePriority=Speed
  Prelookup Alpha : PreLookup  BreakpointsData=AC.Aero.CL.alpha_dat.alpha  ExtrapMethod=Linear
  Prelookup Beta : PreLookup  BreakpointsData=AC.Aero.CL.alpha_dat.beta  ExtrapMethod=Linear
  Out : Outport
  wires:
  Cmdf_l Lookup/1 -> Cmdf_l/2
  Prelookup Alpha/2 -> Cmdf_l Lookup/2
  Bus Selector4/2 -> Prelookup Alpha/1  "<alpha_rad>"
  Bus Selector4/3 -> Prelookup Beta/1  "<beta_rad>"
  Prelookup Alpha/1 -> Cmdf_l Lookup/1
  Prelookup Beta/2 -> Cmdf_l Lookup/4
  Prelookup Beta/1 -> Cmdf_l Lookup/3
  In/1 -> Bus Selector4/1
  Bus Selector4/1 -> Cmdf_l/1  "<l_flap_rad>"
  Cmdf_l/1 -> Out/1

== system Aero_UltraStick25e/Pitch Moment Coefficient/Cmdf_r ==
  In : Inport
  Bus Selector4 : BusSelector  OutputSignals=Actuator States.CtrlSurf.r_flap_rad,WindAxesParams.alpha_rad,WindAxesParams.beta_rad
  Cmdf_r : Product
  Cmdf_r Lookup : Interpolation_n-D  Table=AC.Aero.Cm.dflap_dat.data  InternalRulePriority=Speed
  Prelookup Alpha : PreLookup  BreakpointsData=AC.Aero.CL.alpha_dat.alpha  ExtrapMethod=Linear
  Prelookup Beta : PreLookup  BreakpointsData=AC.Aero.CL.alpha_dat.beta  ExtrapMethod=Linear
  Out : Outport
  wires:
  Cmdf_r Lookup/1 -> Cmdf_r/2
  Prelookup Alpha/2 -> Cmdf_r Lookup/2
  Bus Selector4/2 -> Prelookup Alpha/1  "<alpha_rad>"
  Bus Selector4/3 -> Prelookup Beta/1  "<beta_rad>"
  Prelookup Alpha/1 -> Cmdf_r Lookup/1
  Prelookup Beta/2 -> Cmdf_r Lookup/4
  Prelookup Beta/1 -> Cmdf_r Lookup/3
  In/1 -> Bus Selector4/1
  Bus Selector4/1 -> Cmdf_r/1  "<r_flap_rad>"
  Cmdf_r/1 -> Out/1

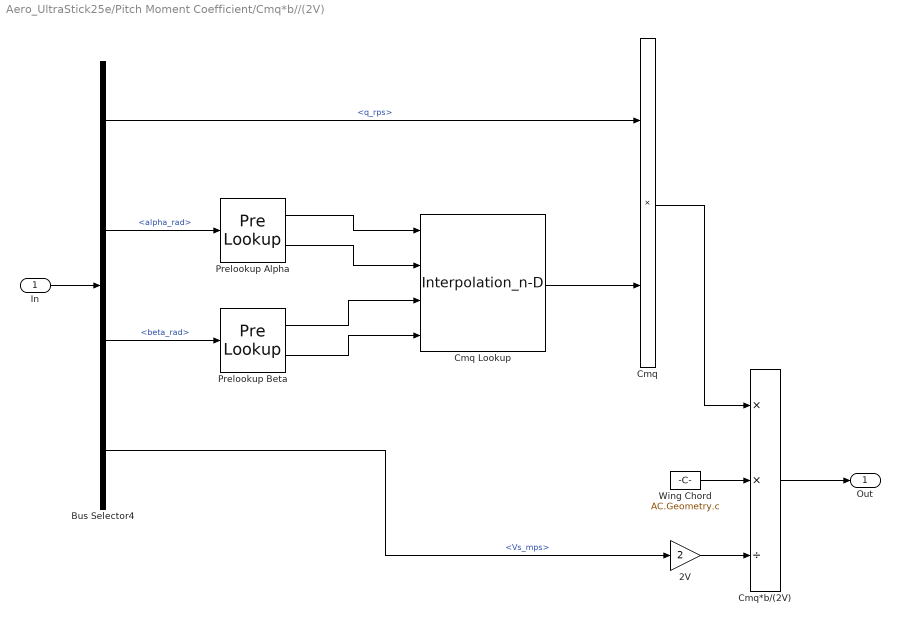
== system Aero_UltraStick25e/Pitch Moment Coefficient/Cmq*b//(2V) ==
  In : Inport
  2V : Gain  Gain=2  SaturateOnIntegerOverflow=on  OutDataTypeStr=Inherit: Same as input  ParamDataTypeStr=Inherit: Same as input
  Bus Selector4 : BusSelector  OutputSignals=AngVel.q_rps,WindAxesParams.alpha_rad,WindAxesParams.beta_rad,WindAxesParams.Vs_mps
  Cmq : Product
  Cmq Lookup : Interpolation_n-D  Table=AC.Aero.Cm.q_dat.data  InternalRulePriority=Speed
  Cmq*b/(2V) : Product  Inputs=**/  SaturateOnIntegerOverflow=on  RndMeth=Zero  InputSameDT=on  OutDataTypeStr=Inherit: Same as first input
  Prelookup Alpha : PreLookup  BreakpointsData=AC.Aero.CL.alpha_dat.alpha  ExtrapMethod=Linear
  Prelookup Beta : PreLookup  BreakpointsData=AC.Aero.CL.alpha_dat.beta  ExtrapMethod=Linear
  Wing Chord : Constant  Value=AC.Geometry.c
  Out : Outport
  wires:
  Bus Selector4/1 -> Cmq/1  "<q_rps>"
  In/1 -> Bus Selector4/1
  Prelookup Beta/1 -> Cmq Lookup/3
  Prelookup Beta/2 -> Cmq Lookup/4
  Prelookup Alpha/1 -> Cmq Lookup/1
  Bus Selector4/3 -> Prelookup Beta/1  "<beta_rad>"
  Bus Selector4/2 -> Prelookup Alpha/1  "<alpha_rad>"
  Prelookup Alpha/2 -> Cmq Lookup/2
  Cmq Lookup/1 -> Cmq/2
  2V/1 -> Cmq*b/(2V)/3
  Wing Chord/1 -> Cmq*b/(2V)/2
  Cmq/1 -> Cmq*b/(2V)/1
  Bus Selector4/4 -> 2V/1  "<Vs_mps>"
  Cmq*b/(2V)/1 -> Out/1

== system Aero_UltraStick25e/Roll Moment Coefficient/Clbeta ==
  In : Inport
  Bus Selector4 : BusSelector  OutputSignals=WindAxesParams.alpha_rad,WindAxesParams.beta_rad
  Clbeta : Product
  Clbeta Lookup : Interpolation_n-D  Table=AC.Aero.Cl.beta_dat.data  InternalRulePriority=Speed
  Prelookup Alpha : PreLookup  BreakpointsData=AC.Aero.CL.alpha_dat.alpha  ExtrapMethod=Linear
  Prelookup Beta : PreLookup  BreakpointsData=AC.Aero.CL.alpha_dat.beta  ExtrapMethod=Linear
  Out : Outport
  wires:
  In/1 -> Bus Selector4/1
  Prelookup Beta/1 -> Clbeta Lookup/3
  Prelookup Beta/2 -> Clbeta Lookup/4
  Prelookup Alpha/1 -> Clbeta Lookup/1
  Bus Selector4/2 -> Clbeta/2, Prelookup Beta/1  "<beta_rad>"
  Bus Selector4/1 -> Prelookup Alpha/1  "<alpha_rad>"
  Prelookup Alpha/2 -> Clbeta Lookup/2
  Clbeta/1 -> Out/1
  Clbeta Lookup/1 -> Clbeta/1

== system Aero_UltraStick25e/Roll Moment Coefficient/Cldail_l ==
  In : Inport
  Bus Selector4 : BusSelector  OutputSignals=Actuator States.CtrlSurf.l_aileron_rad,WindAxesParams.alpha_rad,WindAxesParams.beta_rad
  Cldail_l : Product
  Cldail_l Lookup : Interpolation_n-D  Table=AC.Aero.Cl.dail_dat.data  InternalRulePriority=Speed
  Gain : Gain  Gain=-1
  Prelookup Alpha : PreLookup  BreakpointsData=AC.Aero.CL.alpha_dat.alpha  ExtrapMethod=Linear
  Prelookup Beta : PreLookup  BreakpointsData=AC.Aero.CL.alpha_dat.beta  ExtrapMethod=Linear
  Out : Outport
  wires:
  Cldail_l/1 -> Gain/1
  Cldail_l Lookup/1 -> Cldail_l/2
  Prelookup Alpha/2 -> Cldail_l Lookup/2
  Bus Selector4/2 -> Prelookup Alpha/1  "<alpha_rad>"
  Bus Selector4/3 -> Prelookup Beta/1  "<beta_rad>"
  Prelookup Alpha/1 -> Cldail_l Lookup/1
  Prelookup Beta/2 -> Cldail_l Lookup/4
  Prelookup Beta/1 -> Cldail_l Lookup/3
  In/1 -> Bus Selector4/1
  Bus Selector4/1 -> Cldail_l/1  "<l_aileron_rad>"
  Gain/1 -> Out/1

== system Aero_UltraStick25e/Roll Moment Coefficient/Cldail_r ==
  In : Inport
  Bus Selector4 : BusSelector  OutputSignals=Actuator States.CtrlSurf.r_aileron_rad,WindAxesParams.alpha_rad,WindAxesParams.beta_rad
  Cldail_r : Product
  Cldail_r Lookup : Interpolation_n-D  Table=AC.Aero.Cl.dail_dat.data  InternalRulePriority=Speed
  Prelookup Alpha : PreLookup  BreakpointsData=AC.Aero.CL.alpha_dat.alpha  ExtrapMethod=Linear
  Prelookup Beta : PreLookup  BreakpointsData=AC.Aero.CL.alpha_dat.beta  ExtrapMethod=Linear
  Out : Outport
  wires:
  Cldail_r/1 -> Out/1
  Cldail_r Lookup/1 -> Cldail_r/2
  Prelookup Alpha/2 -> Cldail_r Lookup/2
  Bus Selector4/2 -> Prelookup Alpha/1  "<alpha_rad>"
  Bus Selector4/3 -> Prelookup Beta/1  "<beta_rad>"
  Prelookup Alpha/1 -> Cldail_r Lookup/1
  Prelookup Beta/2 -> Cldail_r Lookup/4
  Prelookup Beta/1 -> Cldail_r Lookup/3
  In/1 -> Bus Selector4/1
  Bus Selector4/1 -> Cldail_r/1  "<r_aileron_rad>"

== system Aero_UltraStick25e/Roll Moment Coefficient/Cldf_l ==
  In : Inport
  Bus Selector4 : BusSelector  OutputSignals=Actuator States.CtrlSurf.l_flap_rad,WindAxesParams.alpha_rad,WindAxesParams.beta_rad
  Cldf_l : Product
  Cldf_l Lookup : Interpolation_n-D  Table=AC.Aero.Cl.dflap_dat.data  InternalRulePriority=Speed
  Gain : Gain  Gain=-1
  Prelookup Alpha : PreLookup  BreakpointsData=AC.Aero.CL.alpha_dat.alpha  ExtrapMethod=Linear
  Prelookup Beta : PreLookup  BreakpointsData=AC.Aero.CL.alpha_dat.beta  ExtrapMethod=Linear
  Out : Outport
  wires:
  Cldf_l/1 -> Gain/1
  Cldf_l Lookup/1 -> Cldf_l/2
  Prelookup Alpha/2 -> Cldf_l Lookup/2
  Bus Selector4/2 -> Prelookup Alpha/1  "<alpha_rad>"
  Bus Selector4/3 -> Prelookup Beta/1  "<beta_rad>"
  Prelookup Alpha/1 -> Cldf_l Lookup/1
  Prelookup Beta/2 -> Cldf_l Lookup/4
  Prelookup Beta/1 -> Cldf_l Lookup/3
  In/1 -> Bus Selector4/1
  Bus Selector4/1 -> Cldf_l/1  "<l_flap_rad>"
  Gain/1 -> Out/1

== system Aero_UltraStick25e/Roll Moment Coefficient/Cldf_r ==
  In : Inport
  Bus Selector4 : BusSelector  OutputSignals=Actuator States.CtrlSurf.r_flap_rad,WindAxesParams.alpha_rad,WindAxesParams.beta_rad
  Cldf_r : Product
  Cldf_r Lookup : Interpolation_n-D  Table=AC.Aero.Cl.dflap_dat.data  InternalRulePriority=Speed
  Prelookup Alpha : PreLookup  BreakpointsData=AC.Aero.CL.alpha_dat.alpha  ExtrapMethod=Linear
  Prelookup Beta : PreLookup  BreakpointsData=AC.Aero.CL.alpha_dat.beta  ExtrapMethod=Linear
  Out : Outport
  wires:
  Cldf_r Lookup/1 -> Cldf_r/2
  Prelookup Alpha/2 -> Cldf_r Lookup/2
  Bus Selector4/2 -> Prelookup Alpha/1  "<alpha_rad>"
  Bus Selector4/3 -> Prelookup Beta/1  "<beta_rad>"
  Prelookup Alpha/1 -> Cldf_r Lookup/1
  Prelookup Beta/2 -> Cldf_r Lookup/4
  Prelookup Beta/1 -> Cldf_r Lookup/3
  In/1 -> Bus Selector4/1
  Bus Selector4/1 -> Cldf_r/1  "<r_flap_rad>"
  Cldf_r/1 -> Out/1

== system Aero_UltraStick25e/Roll Moment Coefficient/Cldrud ==
  In : Inport
  Bus Selector4 : BusSelector  OutputSignals=Actuator States.CtrlSurf.rudder_rad,WindAxesParams.alpha_rad,WindAxesParams.beta_rad
  Cldrud : Product
  Cldrud Lookup : Interpolation_n-D  Table=AC.Aero.Cl.drud_dat.data  InternalRulePriority=Speed
  Prelookup Alpha : PreLookup  BreakpointsData=AC.Aero.CL.alpha_dat.alpha  ExtrapMethod=Linear
  Prelookup Beta : PreLookup  BreakpointsData=AC.Aero.CL.alpha_dat.beta  ExtrapMethod=Linear
  Out : Outport
  wires:
  Cldrud Lookup/1 -> Cldrud/2
  Prelookup Alpha/2 -> Cldrud Lookup/2
  Bus Selector4/2 -> Prelookup Alpha/1  "<alpha_rad>"
  Bus Selector4/3 -> Prelookup Beta/1  "<beta_rad>"
  Prelookup Alpha/1 -> Cldrud Lookup/1
  Prelookup Beta/2 -> Cldrud Lookup/4
  Prelookup Beta/1 -> Cldrud Lookup/3
  In/1 -> Bus Selector4/1
  Bus Selector4/1 -> Cldrud/1  "<rudder_rad>"
  Cldrud/1 -> Out/1

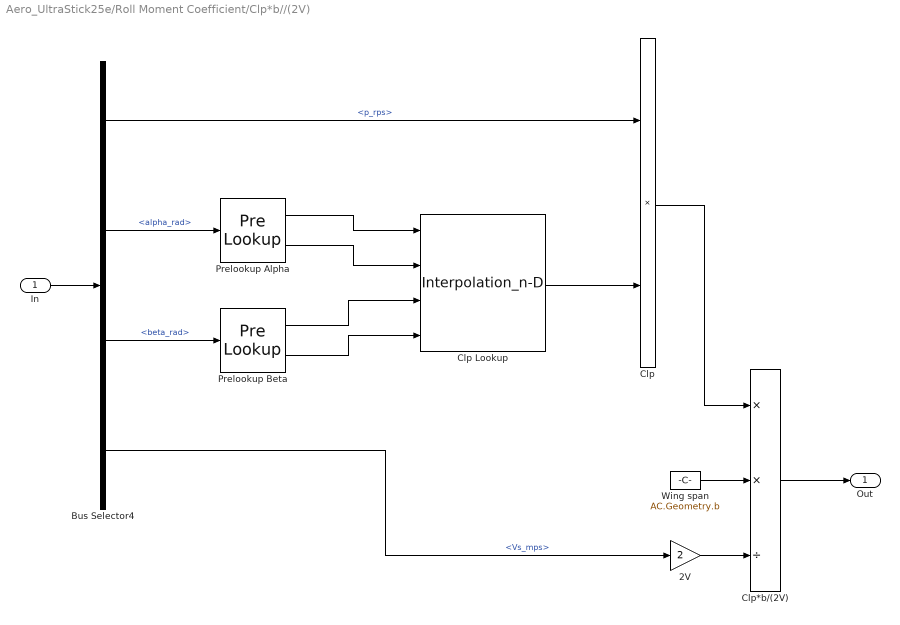
== system Aero_UltraStick25e/Roll Moment Coefficient/Clp*b//(2V) ==
  In : Inport
  2V : Gain  Gain=2  SaturateOnIntegerOverflow=on  OutDataTypeStr=Inherit: Same as input  ParamDataTypeStr=Inherit: Same as input
  Bus Selector4 : BusSelector  OutputSignals=AngVel.p_rps,WindAxesParams.alpha_rad,WindAxesParams.beta_rad,WindAxesParams.Vs_mps
  Clp : Product
  Clp Lookup : Interpolation_n-D  Table=AC.Aero.Cl.p_dat.data  InternalRulePriority=Speed
  Clp*b/(2V) : Product  Inputs=**/  SaturateOnIntegerOverflow=on  RndMeth=Zero  InputSameDT=on  OutDataTypeStr=Inherit: Same as first input
  Prelookup Alpha : PreLookup  BreakpointsData=AC.Aero.CL.alpha_dat.alpha  ExtrapMethod=Linear
  Prelookup Beta : PreLookup  BreakpointsData=AC.Aero.CL.alpha_dat.beta  ExtrapMethod=Linear
  Wing span : Constant  Value=AC.Geometry.b
  Out : Outport
  wires:
  Bus Selector4/1 -> Clp/1  "<p_rps>"
  In/1 -> Bus Selector4/1
  Prelookup Beta/1 -> Clp Lookup/3
  Prelookup Beta/2 -> Clp Lookup/4
  Prelookup Alpha/1 -> Clp Lookup/1
  Bus Selector4/3 -> Prelookup Beta/1  "<beta_rad>"
  Bus Selector4/2 -> Prelookup Alpha/1  "<alpha_rad>"
  Prelookup Alpha/2 -> Clp Lookup/2
  Clp Lookup/1 -> Clp/2
  2V/1 -> Clp*b/(2V)/3
  Wing span/1 -> Clp*b/(2V)/2
  Clp/1 -> Clp*b/(2V)/1
  Bus Selector4/4 -> 2V/1  "<Vs_mps>"
  Clp*b/(2V)/1 -> Out/1

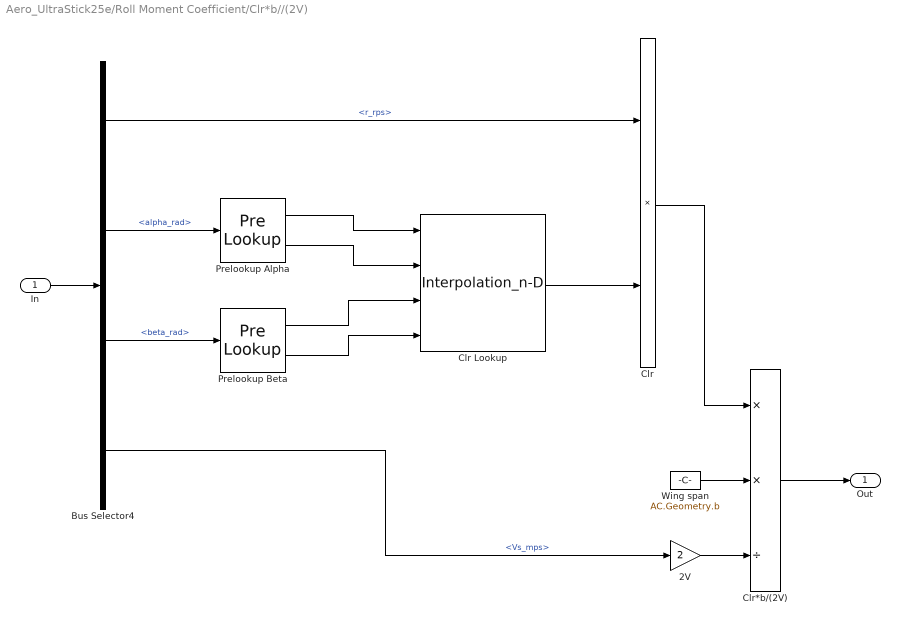
== system Aero_UltraStick25e/Roll Moment Coefficient/Clr*b//(2V) ==
  In : Inport
  2V : Gain  Gain=2  SaturateOnIntegerOverflow=on  OutDataTypeStr=Inherit: Same as input  ParamDataTypeStr=Inherit: Same as input
  Bus Selector4 : BusSelector  OutputSignals=AngVel.r_rps,WindAxesParams.alpha_rad,WindAxesParams.beta_rad,WindAxesParams.Vs_mps
  Clr : Product
  Clr Lookup : Interpolation_n-D  Table=AC.Aero.Cl.r_dat.data  InternalRulePriority=Speed
  Clr*b/(2V) : Product  Inputs=**/  SaturateOnIntegerOverflow=on  RndMeth=Zero  InputSameDT=on  OutDataTypeStr=Inherit: Same as first input
  Prelookup Alpha : PreLookup  BreakpointsData=AC.Aero.CL.alpha_dat.alpha  ExtrapMethod=Linear
  Prelookup Beta : PreLookup  BreakpointsData=AC.Aero.CL.alpha_dat.beta  ExtrapMethod=Linear
  Wing span : Constant  Value=AC.Geometry.b
  Out : Outport
  wires:
  Bus Selector4/1 -> Clr/1  "<r_rps>"
  In/1 -> Bus Selector4/1
  Prelookup Beta/1 -> Clr Lookup/3
  Prelookup Beta/2 -> Clr Lookup/4
  Prelookup Alpha/1 -> Clr Lookup/1
  Bus Selector4/3 -> Prelookup Beta/1  "<beta_rad>"
  Bus Selector4/2 -> Prelookup Alpha/1  "<alpha_rad>"
  Prelookup Alpha/2 -> Clr Lookup/2
  Clr Lookup/1 -> Clr/2
  2V/1 -> Clr*b/(2V)/3
  Wing span/1 -> Clr*b/(2V)/2
  Clr/1 -> Clr*b/(2V)/1
  Bus Selector4/4 -> 2V/1  "<Vs_mps>"
  Clr*b/(2V)/1 -> Out/1

== system Aero_UltraStick25e/Side Force Coefficient/CYwbeta ==
  In : Inport
  Bus Selector4 : BusSelector  OutputSignals=WindAxesParams.alpha_rad,WindAxesParams.beta_rad
  CYwbeta : Product
  CYwbeta Lookup : Interpolation_n-D  Table=AC.Aero.CYw.beta_dat.data  InternalRulePriority=Speed
  Prelookup Alpha : PreLookup  BreakpointsData=AC.Aero.CL.alpha_dat.alpha  ExtrapMethod=Linear
  Prelookup Beta : PreLookup  BreakpointsData=AC.Aero.CL.alpha_dat.beta  ExtrapMethod=Linear
  Out : Outport
  wires:
  In/1 -> Bus Selector4/1
  Prelookup Beta/1 -> CYwbeta Lookup/3
  Prelookup Beta/2 -> CYwbeta Lookup/4
  Prelookup Alpha/1 -> CYwbeta Lookup/1
  Bus Selector4/2 -> CYwbeta/2, Prelookup Beta/1  "<beta_rad>"
  Bus Selector4/1 -> Prelookup Alpha/1  "<alpha_rad>"
  Prelookup Alpha/2 -> CYwbeta Lookup/2
  CYwbeta/1 -> Out/1
  CYwbeta Lookup/1 -> CYwbeta/1

== system Aero_UltraStick25e/Side Force Coefficient/CYwdail_l ==
  In : Inport
  Bus Selector4 : BusSelector  OutputSignals=Actuator States.CtrlSurf.l_aileron_rad,WindAxesParams.alpha_rad,WindAxesParams.beta_rad
  CYwdail_l : Product
  CYwdail_l Lookup : Interpolation_n-D  Table=AC.Aero.CYw.dail_dat.data  InternalRulePriority=Speed
  Prelookup Alpha : PreLookup  BreakpointsData=AC.Aero.CL.alpha_dat.alpha  ExtrapMethod=Linear
  Prelookup Beta : PreLookup  BreakpointsData=AC.Aero.CL.alpha_dat.beta  ExtrapMethod=Linear
  Out : Outport
  wires:
  CYwdail_l/1 -> Out/1
  CYwdail_l Lookup/1 -> CYwdail_l/2
  Prelookup Alpha/2 -> CYwdail_l Lookup/2
  Bus Selector4/2 -> Prelookup Alpha/1  "<alpha_rad>"
  Bus Selector4/3 -> Prelookup Beta/1  "<beta_rad>"
  Prelookup Alpha/1 -> CYwdail_l Lookup/1
  Prelookup Beta/2 -> CYwdail_l Lookup/4
  Prelookup Beta/1 -> CYwdail_l Lookup/3
  In/1 -> Bus Selector4/1
  Bus Selector4/1 -> CYwdail_l/1  "<l_aileron_rad>"

== system Aero_UltraStick25e/Side Force Coefficient/CYwdrud ==
  In : Inport
  Bus Selector4 : BusSelector  OutputSignals=Actuator States.CtrlSurf.rudder_rad,WindAxesParams.alpha_rad,WindAxesParams.beta_rad
  CYwdrud : Product
  CYwdrud Lookup : Interpolation_n-D  Table=AC.Aero.CYw.drud_dat.data  InternalRulePriority=Speed
  Prelookup Alpha : PreLookup  BreakpointsData=AC.Aero.CL.alpha_dat.alpha  ExtrapMethod=Linear
  Prelookup Beta : PreLookup  BreakpointsData=AC.Aero.CL.alpha_dat.beta  ExtrapMethod=Linear
  Out : Outport
  wires:
  CYwdrud Lookup/1 -> CYwdrud/2
  Prelookup Alpha/2 -> CYwdrud Lookup/2
  Bus Selector4/2 -> Prelookup Alpha/1  "<alpha_rad>"
  Bus Selector4/3 -> Prelookup Beta/1  "<beta_rad>"
  Prelookup Alpha/1 -> CYwdrud Lookup/1
  Prelookup Beta/2 -> CYwdrud Lookup/4
  Prelookup Beta/1 -> CYwdrud Lookup/3
  In/1 -> Bus Selector4/1
  Bus Selector4/1 -> CYwdrud/1  "<rudder_rad>"
  CYwdrud/1 -> Out/1

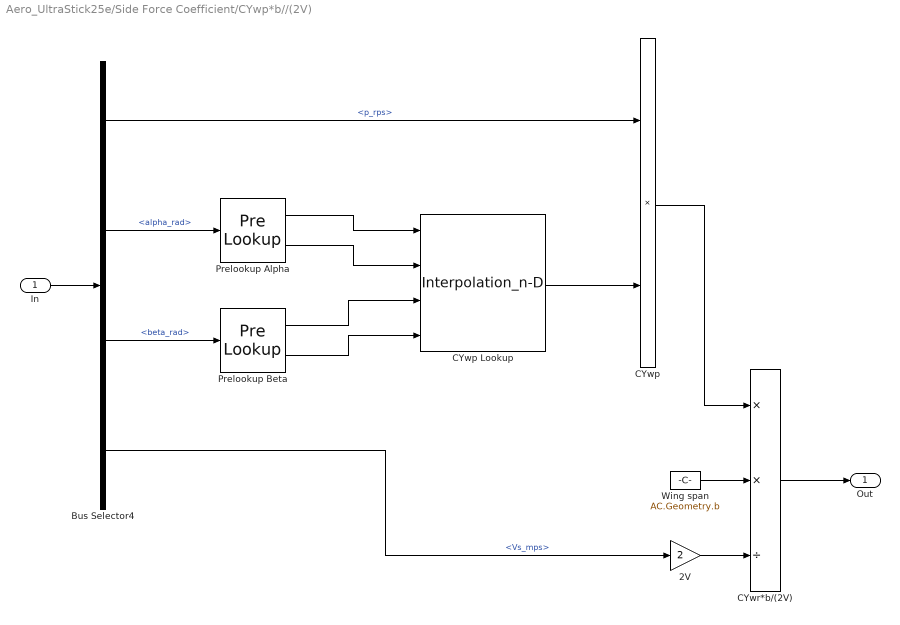
== system Aero_UltraStick25e/Side Force Coefficient/CYwp*b//(2V) ==
  In : Inport
  2V : Gain  Gain=2  SaturateOnIntegerOverflow=on  OutDataTypeStr=Inherit: Same as input  ParamDataTypeStr=Inherit: Same as input
  Bus Selector4 : BusSelector  OutputSignals=AngVel.p_rps,WindAxesParams.alpha_rad,WindAxesParams.beta_rad,WindAxesParams.Vs_mps
  CYwp : Product
  CYwp Lookup : Interpolation_n-D  Table=AC.Aero.CYw.p_dat.data  InternalRulePriority=Speed
  CYwr*b/(2V) : Product  Inputs=**/  SaturateOnIntegerOverflow=on  RndMeth=Zero  InputSameDT=on  OutDataTypeStr=Inherit: Same as first input
  Prelookup Alpha : PreLookup  BreakpointsData=AC.Aero.CL.alpha_dat.alpha  ExtrapMethod=Linear
  Prelookup Beta : PreLookup  BreakpointsData=AC.Aero.CL.alpha_dat.beta  ExtrapMethod=Linear
  Wing span : Constant  Value=AC.Geometry.b
  Out : Outport
  wires:
  Bus Selector4/1 -> CYwp/1  "<p_rps>"
  In/1 -> Bus Selector4/1
  Prelookup Beta/1 -> CYwp Lookup/3
  Prelookup Beta/2 -> CYwp Lookup/4
  Prelookup Alpha/1 -> CYwp Lookup/1
  Bus Selector4/3 -> Prelookup Beta/1  "<beta_rad>"
  Bus Selector4/2 -> Prelookup Alpha/1  "<alpha_rad>"
  Prelookup Alpha/2 -> CYwp Lookup/2
  CYwp Lookup/1 -> CYwp/2
  2V/1 -> CYwr*b/(2V)/3
  Wing span/1 -> CYwr*b/(2V)/2
  CYwp/1 -> CYwr*b/(2V)/1
  Bus Selector4/4 -> 2V/1  "<Vs_mps>"
  CYwr*b/(2V)/1 -> Out/1

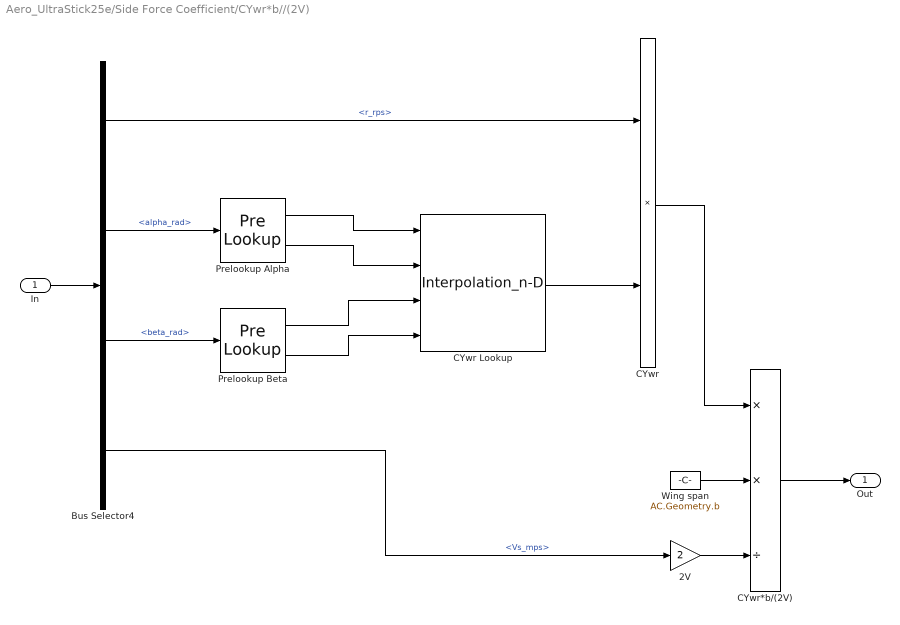
== system Aero_UltraStick25e/Side Force Coefficient/CYwr*b//(2V) ==
  In : Inport
  2V : Gain  Gain=2  SaturateOnIntegerOverflow=on  OutDataTypeStr=Inherit: Same as input  ParamDataTypeStr=Inherit: Same as input
  Bus Selector4 : BusSelector  OutputSignals=AngVel.r_rps,WindAxesParams.alpha_rad,WindAxesParams.beta_rad,WindAxesParams.Vs_mps
  CYwr : Product
  CYwr Lookup : Interpolation_n-D  Table=AC.Aero.CYw.r_dat.data  InternalRulePriority=Speed
  CYwr*b/(2V) : Product  Inputs=**/  SaturateOnIntegerOverflow=on  RndMeth=Zero  InputSameDT=on  OutDataTypeStr=Inherit: Same as first input
  Prelookup Alpha : PreLookup  BreakpointsData=AC.Aero.CL.alpha_dat.alpha  ExtrapMethod=Linear
  Prelookup Beta : PreLookup  BreakpointsData=AC.Aero.CL.alpha_dat.beta  ExtrapMethod=Linear
  Wing span : Constant  Value=AC.Geometry.b
  Out : Outport
  wires:
  Bus Selector4/1 -> CYwr/1  "<r_rps>"
  In/1 -> Bus Selector4/1
  Prelookup Beta/1 -> CYwr Lookup/3
  Prelookup Beta/2 -> CYwr Lookup/4
  Prelookup Alpha/1 -> CYwr Lookup/1
  Bus Selector4/3 -> Prelookup Beta/1  "<beta_rad>"
  Bus Selector4/2 -> Prelookup Alpha/1  "<alpha_rad>"
  Prelookup Alpha/2 -> CYwr Lookup/2
  CYwr Lookup/1 -> CYwr/2
  2V/1 -> CYwr*b/(2V)/3
  Wing span/1 -> CYwr*b/(2V)/2
  CYwr/1 -> CYwr*b/(2V)/1
  Bus Selector4/4 -> 2V/1  "<Vs_mps>"
  CYwr*b/(2V)/1 -> Out/1

== system Aero_UltraStick25e/Side Force Coefficient/Cwdail_r ==
  In : Inport
  Bus Selector4 : BusSelector  OutputSignals=Actuator States.CtrlSurf.r_aileron_rad,WindAxesParams.alpha_rad,WindAxesParams.beta_rad
  CYwdail_r : Product
  CYwdail_r Lookup : Interpolation_n-D  Table=AC.Aero.CYw.dail_dat.data  InternalRulePriority=Speed
  Gain : Gain  Gain=-1
  Prelookup Alpha : PreLookup  BreakpointsData=AC.Aero.CL.alpha_dat.alpha  ExtrapMethod=Linear
  Prelookup Beta : PreLookup  BreakpointsData=AC.Aero.CL.alpha_dat.beta  ExtrapMethod=Linear
  Out : Outport
  wires:
  CYwdail_r/1 -> Gain/1
  CYwdail_r Lookup/1 -> CYwdail_r/2
  Prelookup Alpha/2 -> CYwdail_r Lookup/2
  Bus Selector4/2 -> Prelookup Alpha/1  "<alpha_rad>"
  Bus Selector4/3 -> Prelookup Beta/1  "<beta_rad>"
  Prelookup Alpha/1 -> CYwdail_r Lookup/1
  Prelookup Beta/2 -> CYwdail_r Lookup/4
  Prelookup Beta/1 -> CYwdail_r Lookup/3
  In/1 -> Bus Selector4/1
  Bus Selector4/1 -> CYwdail_r/1  "<r_aileron_rad>"
  Gain/1 -> Out/1

== system Aero_UltraStick25e/Yaw Moment Coefficient/Cnbeta ==
  In : Inport
  Bus Selector4 : BusSelector  OutputSignals=WindAxesParams.alpha_rad,WindAxesParams.beta_rad
  Cnbeta : Product
  Cnbeta Lookup : Interpolation_n-D  Table=AC.Aero.Cn.beta_dat.data  InternalRulePriority=Speed
  Prelookup Alpha : PreLookup  BreakpointsData=AC.Aero.CL.alpha_dat.alpha  ExtrapMethod=Linear
  Prelookup Beta : PreLookup  BreakpointsData=AC.Aero.CL.alpha_dat.beta  ExtrapMethod=Linear
  Out : Outport
  wires:
  In/1 -> Bus Selector4/1
  Prelookup Beta/1 -> Cnbeta Lookup/3
  Prelookup Beta/2 -> Cnbeta Lookup/4
  Prelookup Alpha/1 -> Cnbeta Lookup/1
  Bus Selector4/2 -> Cnbeta/2, Prelookup Beta/1  "<beta_rad>"
  Bus Selector4/1 -> Prelookup Alpha/1  "<alpha_rad>"
  Prelookup Alpha/2 -> Cnbeta Lookup/2
  Cnbeta/1 -> Out/1
  Cnbeta Lookup/1 -> Cnbeta/1

== system Aero_UltraStick25e/Yaw Moment Coefficient/Cndail_l ==
  In : Inport
  Bus Selector4 : BusSelector  OutputSignals=Actuator States.CtrlSurf.l_aileron_rad,WindAxesParams.alpha_rad,WindAxesParams.beta_rad
  Cndail_l : Product
  Cndail_l Lookup : Interpolation_n-D  Table=AC.Aero.Cn.dail_dat.data  InternalRulePriority=Speed
  Gain : Gain  Gain=-1
  Prelookup Alpha : PreLookup  BreakpointsData=AC.Aero.CL.alpha_dat.alpha  ExtrapMethod=Linear
  Prelookup Beta : PreLookup  BreakpointsData=AC.Aero.CL.alpha_dat.beta  ExtrapMethod=Linear
  Out : Outport
  wires:
  Cndail_l/1 -> Gain/1
  Cndail_l Lookup/1 -> Cndail_l/2
  Prelookup Alpha/2 -> Cndail_l Lookup/2
  Bus Selector4/2 -> Prelookup Alpha/1  "<alpha_rad>"
  Bus Selector4/3 -> Prelookup Beta/1  "<beta_rad>"
  Prelookup Alpha/1 -> Cndail_l Lookup/1
  Prelookup Beta/2 -> Cndail_l Lookup/4
  Prelookup Beta/1 -> Cndail_l Lookup/3
  In/1 -> Bus Selector4/1
  Bus Selector4/1 -> Cndail_l/1  "<l_aileron_rad>"
  Gain/1 -> Out/1

== system Aero_UltraStick25e/Yaw Moment Coefficient/Cndail_r ==
  In : Inport
  Bus Selector4 : BusSelector  OutputSignals=Actuator States.CtrlSurf.r_aileron_rad,WindAxesParams.alpha_rad,WindAxesParams.beta_rad
  Cndail_r : Product
  Cndail_r Lookup : Interpolation_n-D  Table=AC.Aero.Cn.dail_dat.data  InternalRulePriority=Speed
  Prelookup Alpha : PreLookup  BreakpointsData=AC.Aero.CL.alpha_dat.alpha  ExtrapMethod=Linear
  Prelookup Beta : PreLookup  BreakpointsData=AC.Aero.CL.alpha_dat.beta  ExtrapMethod=Linear
  Out : Outport
  wires:
  Cndail_r/1 -> Out/1
  Cndail_r Lookup/1 -> Cndail_r/2
  Prelookup Alpha/2 -> Cndail_r Lookup/2
  Bus Selector4/2 -> Prelookup Alpha/1  "<alpha_rad>"
  Bus Selector4/3 -> Prelookup Beta/1  "<beta_rad>"
  Prelookup Alpha/1 -> Cndail_r Lookup/1
  Prelookup Beta/2 -> Cndail_r Lookup/4
  Prelookup Beta/1 -> Cndail_r Lookup/3
  In/1 -> Bus Selector4/1
  Bus Selector4/1 -> Cndail_r/1  "<r_aileron_rad>"

== system Aero_UltraStick25e/Yaw Moment Coefficient/Cndf_l ==
  In : Inport
  Bus Selector4 : BusSelector  OutputSignals=Actuator States.CtrlSurf.l_flap_rad,WindAxesParams.alpha_rad,WindAxesParams.beta_rad
  Cndf_l : Product
  Cndf_l Lookup : Interpolation_n-D  Table=AC.Aero.Cn.dflap_dat.data  InternalRulePriority=Speed
  Gain : Gain  Gain=-1
  Prelookup Alpha : PreLookup  BreakpointsData=AC.Aero.CL.alpha_dat.alpha  ExtrapMethod=Linear
  Prelookup Beta : PreLookup  BreakpointsData=AC.Aero.CL.alpha_dat.beta  ExtrapMethod=Linear
  Out : Outport
  wires:
  Cndf_l/1 -> Gain/1
  Cndf_l Lookup/1 -> Cndf_l/2
  Prelookup Alpha/2 -> Cndf_l Lookup/2
  Bus Selector4/2 -> Prelookup Alpha/1  "<alpha_rad>"
  Bus Selector4/3 -> Prelookup Beta/1  "<beta_rad>"
  Prelookup Alpha/1 -> Cndf_l Lookup/1
  Prelookup Beta/2 -> Cndf_l Lookup/4
  Prelookup Beta/1 -> Cndf_l Lookup/3
  In/1 -> Bus Selector4/1
  Bus Selector4/1 -> Cndf_l/1  "<l_flap_rad>"
  Gain/1 -> Out/1

== system Aero_UltraStick25e/Yaw Moment Coefficient/Cndf_r ==
  In : Inport
  Bus Selector4 : BusSelector  OutputSignals=Actuator States.CtrlSurf.r_flap_rad,WindAxesParams.alpha_rad,WindAxesParams.beta_rad
  Cndf_r : Product
  Cndf_r Lookup : Interpolation_n-D  Table=AC.Aero.Cn.dflap_dat.data  InternalRulePriority=Speed
  Prelookup Alpha : PreLookup  BreakpointsData=AC.Aero.CL.alpha_dat.alpha  ExtrapMethod=Linear
  Prelookup Beta : PreLookup  BreakpointsData=AC.Aero.CL.alpha_dat.beta  ExtrapMethod=Linear
  Out : Outport
  wires:
  Cndf_r Lookup/1 -> Cndf_r/2
  Prelookup Alpha/2 -> Cndf_r Lookup/2
  Bus Selector4/2 -> Prelookup Alpha/1  "<alpha_rad>"
  Bus Selector4/3 -> Prelookup Beta/1  "<beta_rad>"
  Prelookup Alpha/1 -> Cndf_r Lookup/1
  Prelookup Beta/2 -> Cndf_r Lookup/4
  Prelookup Beta/1 -> Cndf_r Lookup/3
  In/1 -> Bus Selector4/1
  Bus Selector4/1 -> Cndf_r/1  "<r_flap_rad>"
  Cndf_r/1 -> Out/1

== system Aero_UltraStick25e/Yaw Moment Coefficient/Cndrud ==
  In : Inport
  Bus Selector4 : BusSelector  OutputSignals=Actuator States.CtrlSurf.rudder_rad,WindAxesParams.alpha_rad,WindAxesParams.beta_rad
  Cndrud : Product
  Cndrud Lookup : Interpolation_n-D  Table=AC.Aero.Cn.drud_dat.data  InternalRulePriority=Speed
  Prelookup Alpha : PreLookup  BreakpointsData=AC.Aero.CL.alpha_dat.alpha  ExtrapMethod=Linear
  Prelookup Beta : PreLookup  BreakpointsData=AC.Aero.CL.alpha_dat.beta  ExtrapMethod=Linear
  Out : Outport
  wires:
  Cndrud Lookup/1 -> Cndrud/2
  Prelookup Alpha/2 -> Cndrud Lookup/2
  Bus Selector4/2 -> Prelookup Alpha/1  "<alpha_rad>"
  Bus Selector4/3 -> Prelookup Beta/1  "<beta_rad>"
  Prelookup Alpha/1 -> Cndrud Lookup/1
  Prelookup Beta/2 -> Cndrud Lookup/4
  Prelookup Beta/1 -> Cndrud Lookup/3
  In/1 -> Bus Selector4/1
  Bus Selector4/1 -> Cndrud/1  "<rudder_rad>"
  Cndrud/1 -> Out/1

== system Aero_UltraStick25e/Yaw Moment Coefficient/Cnp*b//(2V) ==
  In : Inport
  2V : Gain  Gain=2  SaturateOnIntegerOverflow=on  OutDataTypeStr=Inherit: Same as input  ParamDataTypeStr=Inherit: Same as input
  Bus Selector4 : BusSelector  OutputSignals=AngVel.p_rps,WindAxesParams.alpha_rad,WindAxesParams.beta_rad,WindAxesParams.Vs_mps
  Cnp : Product
  Cnp Lookup : Interpolation_n-D  Table=AC.Aero.Cn.p_dat.data  InternalRulePriority=Speed
  Cnp*b/(2V) : Product  Inputs=**/  SaturateOnIntegerOverflow=on  RndMeth=Zero  InputSameDT=on  OutDataTypeStr=Inherit: Same as first input
  Prelookup Alpha : PreLookup  BreakpointsData=AC.Aero.CL.alpha_dat.alpha  ExtrapMethod=Linear
  Prelookup Beta : PreLookup  BreakpointsData=AC.Aero.CL.alpha_dat.beta  ExtrapMethod=Linear
  Wing span : Constant  Value=AC.Geometry.b
  Out : Outport
  wires:
  Bus Selector4/1 -> Cnp/1  "<p_rps>"
  In/1 -> Bus Selector4/1
  Prelookup Beta/1 -> Cnp Lookup/3
  Prelookup Beta/2 -> Cnp Lookup/4
  Prelookup Alpha/1 -> Cnp Lookup/1
  Bus Selector4/3 -> Prelookup Beta/1  "<beta_rad>"
  Bus Selector4/2 -> Prelookup Alpha/1  "<alpha_rad>"
  Prelookup Alpha/2 -> Cnp Lookup/2
  Cnp Lookup/1 -> Cnp/2
  2V/1 -> Cnp*b/(2V)/3
  Wing span/1 -> Cnp*b/(2V)/2
  Cnp/1 -> Cnp*b/(2V)/1
  Bus Selector4/4 -> 2V/1  "<Vs_mps>"
  Cnp*b/(2V)/1 -> Out/1
